simulink library "dma_utils_lib"  (R2023b)
settings: Solver=VariableStepAuto  StartTime=0.0  StopTime=10.0  RelTol=1e-3
libraries: hdlsllib x7, simulink x2
settings Model: Creator=promero  LastModifiedBy=promero

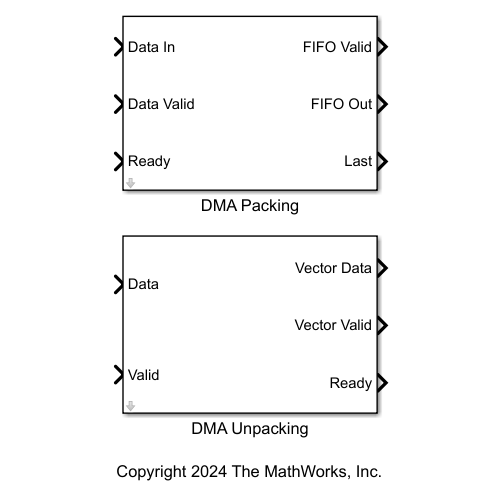
[thumbnail: Simulink's stored preview of the top-level diagram]
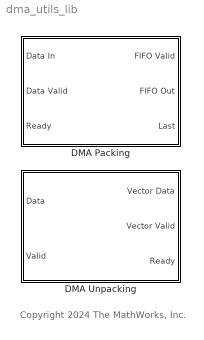
== system dma_utils_lib ==
  note: Copyright 2024 The MathWorks, Inc.
  DMA Packing : Subsystem  mask(DMA Packing){oversampling=1, vectorSize=11, timeFactor=11}
      mask prompts: vectorSize "Vector size"; timeFactor "Sample time factor"
      mask help:
      | This block packs vector data and creates a DMA frame of the same size, ready to connect with the corresponding AXI-Stream ports. It enables two fundamental modes of operation:
      |
      | 1) Buffering data for FPGA-rate logging (frame mode)
      | If you want to buffer data at FPGA model rate to enable signal logging at full FPGA resolution and pass the data frame to the CPU, set the Oversampling value equal to the FPGA to CPU frequency ratio. Set the sample time factor to 1, and adjust the vector size accordingly.
      |
      | 2) Fast FPGA to CPU data transfer at CPU-rate (sample mode)
      | Set Oversample value to 1 and adjust the vector size according to the data size.
      | Set sample time factor to 1, if the FPGA model rate is slower than the FPGA base rate. Otherwise (if you are packing DMA data at the FPGA base rate), set it to the same value than the frame size to downsample the vector data by that factor.
      mask DialogControl ParameterGroupVar Prompt: DMA Data
      mask DialogControl Container3 Prompt: FPGA to CPU Logging
  DMA Unpacking : Subsystem  mask(DMA Unpacking){frameSize=10}
      mask prompts: frameSize "Frame / Vector size"
      mask help: This block unpacks a DMA frame into vector data of the same size, ready to connect with the corresponding AXI-Stream ports.

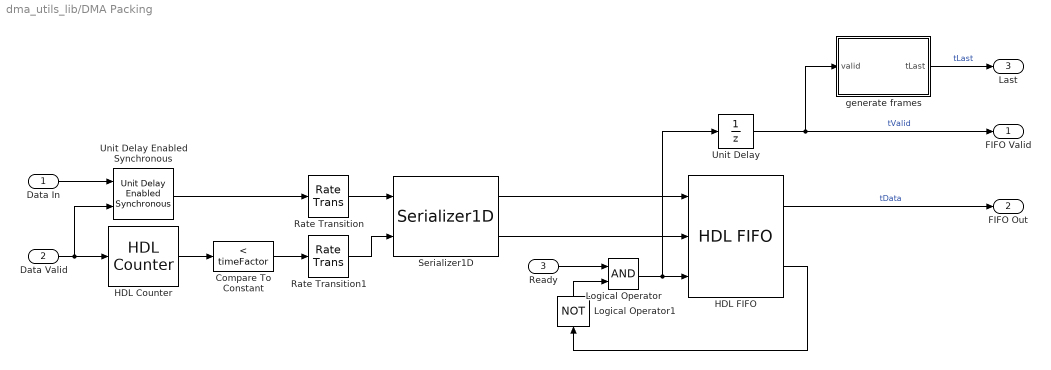
== system dma_utils_lib/DMA Packing ==
  Data In : Inport  OutDataTypeStr=uint32
  Data Valid : Inport  Port=2
  Ready : Inport  Port=3
  Compare To Constant : simulink/Logic and Bit Operations/Compare To Constant  relop=<  const=timeFactor  OutDataTypeStr=boolean
  HDL Counter : hdlsllib/Sources/HDL Counter  CountType=Free running  CountInit=0  CountStep=1  CountMax=25  CountFromType=Initial value  CountFrom=0  CountResetPort=on  CountLoadPort=off  CountEnbPort=off  CountDirPort=off  CountHitOutputPort=off  CountDataType=Unsigned  CountWordLen=32  CountFracLen=0  CountSampTime=1
  HDL FIFO : hdlsllib/HDL RAMs/HDL FIFO  fifo_size=max(vectorSize*oversampling,4)  mode=Classic  ratio=1  push_msg=Warning  pop_msg=Warning  show_empty=on  show_full=off  show_num=off  LabelModeActiveChoice_Mode=Classic  rst_port=off
  Logical Operator : Logic  AllPortsSameDT=off  OutDataTypeStr=boolean
  Logical Operator1 : Logic  Operator=NOT  IconShape=distinctive  AllPortsSameDT=off  OutDataTypeStr=boolean
  Rate Transition : RateTransition  OutPortSampleTimeOpt=Multiple of input port sample time  OutPortSampleTimeMultiple=timeFactor
  Rate Transition1 : RateTransition  OutPortSampleTimeOpt=Multiple of input port sample time  OutPortSampleTimeMultiple=timeFactor
  Serializer1D : hdlsllib/HDL Operations/Serializer1D  Ratio=vectorSize  IdleCycles=0  validIn=on  startOut=off  validOut=on  inputDataDimensions=-1  inputSampleTime=-1  inputSignalType=auto
  Unit Delay : UnitDelay  SampleTime=-1  HasFrameUpgradeWarning=on
  Unit Delay Enabled Synchronous : hdlsllib/Discrete/Unit Delay Enabled Synchronous  InitialCondition=0.0  SampleTime=-1
  generate frames : Subsystem
  FIFO Valid : Outport
  FIFO Out : Outport  Port=2
  Last : Outport  Port=3
  wires:
  generate frames/1(tLast) -> Last/1  "tLast"
  Data In/1 -> Unit Delay Enabled Synchronous/1
  Unit Delay Enabled Synchronous/1 -> Rate Transition/1
  Compare To Constant/1 -> Rate Transition1/1
  Data Valid/1 -> HDL Counter/1, Unit Delay Enabled Synchronous/2
  HDL Counter/1 -> Compare To Constant/1
  HDL FIFO/2 -> Logical Operator1/1
  Rate Transition/1 -> Serializer1D/1
  Ready/1 -> Logical Operator/1
  Unit Delay/1 -> FIFO Valid/1, generate frames/1(valid)  "tValid"
  Logical Operator/1 -> Unit Delay/1, HDL FIFO/3
  Serializer1D/1 -> HDL FIFO/1
  Serializer1D/2 -> HDL FIFO/2
  Logical Operator1/1 -> Logical Operator/2
  Rate Transition1/1 -> Serializer1D/2
  HDL FIFO/1 -> FIFO Out/1  "tData"

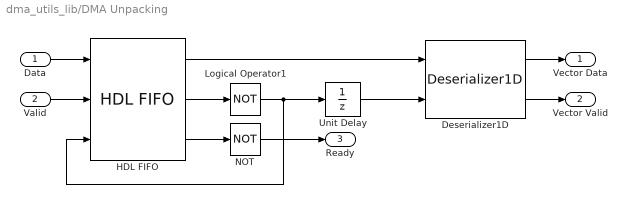
== system dma_utils_lib/DMA Unpacking ==
  Data : Inport  OutDataTypeStr=uint32
  Valid : Inport  Port=2
  Deserializer1D : hdlsllib/HDL Operations/Deserializer1D  Ratio=frameSize  IdleCycles=0  InitialCondition=0  startIn=off  validIn=on  validOut=on  inputDataDimensions=-1  inputSampleTime=-1  inputSignalType=auto
  HDL FIFO : hdlsllib/HDL RAMs/HDL FIFO  fifo_size=max(frameSize,4)  mode=Classic  ratio=1  push_msg=Warning  pop_msg=Warning  show_empty=on  show_full=on  show_num=off  LabelModeActiveChoice_Mode=Classic  rst_port=off
  Logical Operator1 : Logic  Operator=NOT  IconShape=distinctive  AllPortsSameDT=off  OutDataTypeStr=boolean
  NOT : Logic  Operator=NOT  IconShape=distinctive  AllPortsSameDT=off  OutDataTypeStr=boolean
  Unit Delay : UnitDelay  SampleTime=-1  HasFrameUpgradeWarning=on
  Vector Data : Outport
  Vector Valid : Outport  Port=2
  Ready : Outport  Port=3
  wires:
  Unit Delay/1 -> Deserializer1D/2
  Valid/1 -> HDL FIFO/2
  Logical Operator1/1 -> HDL FIFO/3, Unit Delay/1
  Data/1 -> HDL FIFO/1
  NOT/1 -> Ready/1
  HDL FIFO/3 -> NOT/1
  HDL FIFO/1 -> Deserializer1D/1
  HDL FIFO/2 -> Logical Operator1/1
  Deserializer1D/1 -> Vector Data/1
  Deserializer1D/2 -> Vector Valid/1

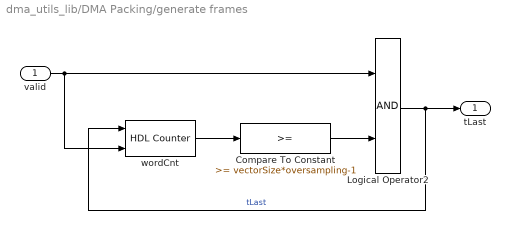
== system dma_utils_lib/DMA Packing/generate frames ==
  valid : Inport
  Compare To Constant : simulink/Logic and Bit Operations/Compare To Constant  relop=>=  const=vectorSize*oversampling-1  OutDataTypeStr=boolean
  Logical Operator2 : Logic  AllPortsSameDT=off  OutDataTypeStr=boolean
  wordCnt : hdlsllib/Sources/HDL Counter  CountType=Free running  CountInit=0  CountStep=1  CountMax=16  CountFromType=Initial value  CountFrom=0  CountResetPort=on  CountLoadPort=off  CountEnbPort=on  CountDirPort=off  CountHitOutputPort=off  CountDataType=Unsigned  CountWordLen=32  CountFracLen=0  CountSampTime=1
  tLast : Outport  VectorParamsAs1DForOutWhenUnconnected=off
  wires:
  Compare To Constant/1 -> Logical Operator2/2
  wordCnt/1 -> Compare To Constant/1
  valid/1 -> Logical Operator2/1, wordCnt/2
  Logical Operator2/1 -> tLast/1, wordCnt/1  "tLast"
